simulink model "s_cd_hmc_v2"  (R2016b)
(part 2 of 43)

      mask prompts: io_dir "I/O direction"; io_delay "I/O delay"; sample_period "Sample period"; names "Bitfield names [msb...lsb]"; bitwidths "Bitfield widths"; bin_pts "Bitfield binary pts"; arith_types "Bitfield types, ufix=0, fix=1, bool=2"; sim_port "Provide sim input/output?"; show_format "Print format string?"
      mask help: A 32-bit software-accessible register. Can be divided into bitfields of varying widths and types using the fields in the block mask.
      mask init:
      | swreg_init(gcb)
      settings: AttributesFormatString=1input:uf32.0 = 32 bits
      mask TypeOptions io_dir: To Processor | From Processor
      mask Callback io_dir:
      | mask_enables = get_param(gcb, 'MaskEnables');
      | mask_names = get_param(gcb, 'MaskNames');
      | if strcmp(get_param(gcb, 'io_dir'), 'To Processor'),
      |     mask_enables{ismember(mask_names, 'sample_period')} = 'off';
      | else
      |     mask_enables{ismember(mask_names, 'sample_period')} = 'on';
      | end
      | set_param(gcb, 'MaskEnables', mask_enables);
  sync : Subsystem  Tag=xps:sw_reg  AncestorBlock=xps_library/software_register  mask(swreg){io_dir=To Processor, io_delay=0, sample_period=1, names=reg, bitwidths=1, bin_pts=0, arith_types=2, sim_port=on, show_format=on}
      mask prompts: io_dir "I/O direction"; io_delay "I/O delay"; sample_period "Sample period"; names "Bitfield names [msb...lsb]"; bitwidths "Bitfield widths"; bin_pts "Bitfield binary pts"; arith_types "Bitfield types, ufix=0, fix=1, bool=2"; sim_port "Provide sim input/output?"; show_format "Print format string?"
      mask help: A 32-bit software-accessible register. Can be divided into bitfields of varying widths and types using the fields in the block mask.
      mask init:
      | swreg_init(gcb)
      settings: AttributesFormatString=1output:b = 1 bits
      mask TypeOptions io_dir: To Processor | From Processor
      mask Callback io_dir:
      | mask_enables = get_param(gcb, 'MaskEnables');
      | mask_names = get_param(gcb, 'MaskNames');
      | if strcmp(get_param(gcb, 'io_dir'), 'To Processor'),
      |     mask_enables{ismember(mask_names, 'sample_period')} = 'off';
      | else
      |     mask_enables{ismember(mask_names, 'sample_period')} = 'on';
      | end
      | set_param(gcb, 'MaskEnables', mask_enables);
  sync_cnt : Subsystem  Tag=xps:sw_reg  AncestorBlock=xps_library/software_register  mask(swreg){io_dir=To Processor, io_delay=0, sample_period=1, names=reg, bitwidths=32, bin_pts=0, arith_types=0, sim_port=on, show_format=on}
      mask prompts: io_dir "I/O direction"; io_delay "I/O delay"; sample_period "Sample period"; names "Bitfield names [msb...lsb]"; bitwidths "Bitfield widths"; bin_pts "Bitfield binary pts"; arith_types "Bitfield types, ufix=0, fix=1, bool=2"; sim_port "Provide sim input/output?"; show_format "Print format string?"
      mask help: A 32-bit software-accessible register. Can be divided into bitfields of varying widths and types using the fields in the block mask.
      mask init:
      | swreg_init(gcb)
      settings: AttributesFormatString=1output:uf32.0 = 32 bits
      mask TypeOptions io_dir: To Processor | From Processor
      mask Callback io_dir:
      | mask_enables = get_param(gcb, 'MaskEnables');
      | mask_names = get_param(gcb, 'MaskNames');
      | if strcmp(get_param(gcb, 'io_dir'), 'To Processor'),
      |     mask_enables{ismember(mask_names, 'sample_period')} = 'off';
      | else
      |     mask_enables{ismember(mask_names, 'sample_period')} = 'on';
      | end
      | set_param(gcb, 'MaskEnables', mask_enables);
  sync_select : Subsystem  Tag=xps:sw_reg  AncestorBlock=xps_library/software register  mask(swreg){io_dir=From Processor, io_delay=0, sample_period=1, names=reg, bitwidths=2, bin_pts=0, arith_types=0, sim_port=on, show_format=on}
      mask prompts: io_dir "I/O direction"; io_delay "I/O delay"; sample_period "Sample period"; names "Bitfield names [msb...lsb]"; bitwidths "Bitfield widths"; bin_pts "Bitfield binary pts"; arith_types "Bitfield types, ufix=0, fix=1, bool=2"; sim_port "Provide sim input/output?"; show_format "Print format string?"
      mask help: A 32-bit software-accessible register. Can be divided into bitfields of varying widths and types using the fields in the block mask.
      mask init:
      | swreg_init(gcb)
      settings: AttributesFormatString=1input:uf2.0 = 2 bits
      mask TypeOptions io_dir: To Processor | From Processor
      mask Callback io_dir:
      | mask_enables = get_param(gcb, 'MaskEnables');
      | mask_names = get_param(gcb, 'MaskNames');
      | if strcmp(get_param(gcb, 'io_dir'), 'To Processor'),
      |     mask_enables{ismember(mask_names, 'sample_period')} = 'off';
      | else
      |     mask_enables{ismember(mask_names, 'sample_period')} = 'on';
      | end
      | set_param(gcb, 'MaskEnables', mask_enables);
  tl_cd0 : Subsystem  mask(timed_latch){n_bits_time=48-(fft_stages+8), n_bits_quantization=fft_stages+8, n_bits_counters=4}
      mask prompts: n_bits_time "Number bits in time to compare"; n_bits_quantization "Time offset from lsb"; n_bits_counters "Bits in status counters"
      mask help:
      | Latches load_value when armed and current_time matches requested time.
      | current_time should be in ADC samples.
      mask init:
      | set_param([gcb,'/status'], 'bitwidths', mat2str([1, repmat(n_bits_counters, 1, 2)]));
      mask Help:
      | When armed, will latch new value when current time matches the time
      | specified. The input time should be in samples and mask settings allow
      | a portion of this to be compared to cater for quantization. Arm and latch
      | counts allow the current state, pending and missed latch events to be
      | determined.
  tl_cd1 : Subsystem  mask(timed_latch){n_bits_time=48-(fft_stages+8), n_bits_quantization=fft_stages+8, n_bits_counters=4}
      mask prompts: n_bits_time "Number bits in time to compare"; n_bits_quantization "Time offset from lsb"; n_bits_counters "Bits in status counters"
      mask help:
      | Latches load_value when armed and current_time matches requested time.
      | current_time should be in ADC samples.
      mask init:
      | set_param([gcb,'/status'], 'bitwidths', mat2str([1, repmat(n_bits_counters, 1, 2)]));
      mask Help:
      | When armed, will latch new value when current time matches the time
      | specified. The input time should be in samples and mask settings allow
      | a portion of this to be compared to cater for quantization. Arm and latch
      | counts allow the current state, pending and missed latch events to be
      | determined.
  tx_metadata : Subsystem  Tag=xps:sw_reg  AncestorBlock=xps_library/software register  mask(swreg){io_dir=From Processor, io_delay=0, sample_period=1, names=[porttx board_id], bitwidths=16, bin_pts=0, arith_types=0, sim_port=on, show_format=on}
      mask prompts: io_dir "I/O direction"; io_delay "I/O delay"; sample_period "Sample period"; names "Bitfield names [msb...lsb]"; bitwidths "Bitfield widths"; bin_pts "Bitfield binary pts"; arith_types "Bitfield types, ufix=0, fix=1, bool=2"; sim_port "Provide sim input/output?"; show_format "Print format string?"
      mask help: A 32-bit software-accessible register. Can be divided into bitfields of varying widths and types using the fields in the block mask.
      mask init:
      | swreg_init(gcb)
      settings: AttributesFormatString=2 inputs:uf16.0,uf16.0 = 32 bits
      mask TypeOptions io_dir: To Processor | From Processor
      mask Callback io_dir:
      | mask_enables = get_param(gcb, 'MaskEnables');
      | mask_names = get_param(gcb, 'MaskNames');
      | if strcmp(get_param(gcb, 'io_dir'), 'To Processor'),
      |     mask_enables{ismember(mask_names, 'sample_period')} = 'off';
      | else
      |     mask_enables{ismember(mask_names, 'sample_period')} = 'on';
      | end
      | set_param(gcb, 'MaskEnables', mask_enables);
  valid80 : Subsystem  Tag=xps:sw_reg  AncestorBlock=xps_library/software_register  mask(swreg){io_dir=To Processor, io_delay=0, sample_period=1, names=reg, bitwidths=1, bin_pts=0, arith_types=2, sim_port=on, show_format=on}
      mask prompts: io_dir "I/O direction"; io_delay "I/O delay"; sample_period "Sample period"; names "Bitfield names [msb...lsb]"; bitwidths "Bitfield widths"; bin_pts "Bitfield binary pts"; arith_types "Bitfield types, ufix=0, fix=1, bool=2"; sim_port "Provide sim input/output?"; show_format "Print format string?"
      mask help: A 32-bit software-accessible register. Can be divided into bitfields of varying widths and types using the fields in the block mask.
      mask init:
      | swreg_init(gcb)
      settings: AttributesFormatString=1output:b = 1 bits
      mask TypeOptions io_dir: To Processor | From Processor
      mask Callback io_dir:
      | mask_enables = get_param(gcb, 'MaskEnables');
      | mask_names = get_param(gcb, 'MaskNames');
      | if strcmp(get_param(gcb, 'io_dir'), 'To Processor'),
      |     mask_enables{ismember(mask_names, 'sample_period')} = 'off';
      | else
      |     mask_enables{ismember(mask_names, 'sample_period')} = 'on';
      | end
      | set_param(gcb, 'MaskEnables', mask_enables);
  valid80_cnt : Subsystem  Tag=xps:sw_reg  AncestorBlock=xps_library/software_register  mask(swreg){io_dir=To Processor, io_delay=0, sample_period=1, names=reg, bitwidths=32, bin_pts=0, arith_types=0, sim_port=on, show_format=on}
      mask prompts: io_dir "I/O direction"; io_delay "I/O delay"; sample_period "Sample period"; names "Bitfield names [msb...lsb]"; bitwidths "Bitfield widths"; bin_pts "Bitfield binary pts"; arith_types "Bitfield types, ufix=0, fix=1, bool=2"; sim_port "Provide sim input/output?"; show_format "Print format string?"
      mask help: A 32-bit software-accessible register. Can be divided into bitfields of varying widths and types using the fields in the block mask.
      mask init:
      | swreg_init(gcb)
      settings: AttributesFormatString=1output:uf32.0 = 32 bits
      mask TypeOptions io_dir: To Processor | From Processor
      mask Callback io_dir:
      | mask_enables = get_param(gcb, 'MaskEnables');
      | mask_names = get_param(gcb, 'MaskNames');
      | if strcmp(get_param(gcb, 'io_dir'), 'To Processor'),
      |     mask_enables{ismember(mask_names, 'sample_period')} = 'off';
      | else
      |     mask_enables{ismember(mask_names, 'sample_period')} = 'on';
      | end
      | set_param(gcb, 'MaskEnables', mask_enables);
  tag scope: cnt_rst=global, dvalid=global, man_sys_rst=global, sync_select=global
  wires:
  Constant/1 -> port0/1(sim_1)
  port0/1(in_reg) -> Delay16/1
  Constant2/1 -> ip0/1(sim_1)
  ip0/1(in_reg) -> Delay15/1
  Constant3/1 -> forty_gbe/8(rx_overrun_ack)
  Constant4/1 -> forty_gbe/7(rx_ack)
  [gbe_rst] -> pipeline102/1(d)
  Delay15/1 -> forty_gbe/4(tx_dest_ip)
  Delay16/1 -> forty_gbe/5(tx_dest_port)
  Concat22/1 -> pipeline29/1(d)
  Concat3/1 -> pipeline27/1(d)
  phase0/1(in_initial) -> Reinterpret2/1
  delta_delay0/1(in_delta) -> Reinterpret1/1
  phase0/2(in_delta) -> Reinterpret3/1
  Reinterpret8/1 -> pipeline56/1(d)
  Reinterpret1/1 -> pipeline55/1(d)
  Reinterpret2/1 -> pipeline54/1(d)
  Reinterpret3/1 -> pipeline53/1(d)
  phase1/1(in_initial) -> Reinterpret5/1
  delta_delay1/1(in_delta) -> Reinterpret4/1
  phase1/2(in_delta) -> Reinterpret6/1
  Reinterpret4/1 -> pipeline51/1(d)
  Reinterpret5/1 -> pipeline50/1(d)
  Reinterpret6/1 -> pipeline49/1(d)
  Reinterpret7/1 -> pipeline52/1(d)
  delay0/1(in_initial) -> Reinterpret8/1
  delay1/1(in_initial) -> Reinterpret7/1
  Constant10/1 -> iptx_base/1(sim_1)
  Constant9/1 -> tx_metadata/1(sim_1)
  Constant13/1 -> tx_metadata/2(sim_2)
  iptx_base/1(in_reg) -> pipeline105/1(d)
  pipeline105/1(q) -> [tx_ip_base]
  tx_metadata/1(in_porttx) -> pipeline106/1(d)
  tx_metadata/2(in_board_id) -> pipeline107/1(d)
  pipeline106/1(q) -> [tx_port]
  pipeline107/1(q) -> [tx_board_id]
  edge_detect4/1(out) -> pipeline5/1(d)
  control1/6(in_cnt_rst) -> edge_detect1/1(in)
  edge_detect1/1(out) -> pipeline14/1(d)
  control1/3(in_gbe_rst) -> pipeline6/1(d)
  control1/1(in_sys_rst) -> pipeline3/1(d)
  pipeline3/1(q) -> [sys_rst]
  pipeline5/1(q) -> [clr_status]
  pipeline6/1(q) -> [gbe_rst]
  pipeline7/1(q) -> [gbe_txen]
  pipeline13/1(q) -> [tvg_adc_en]
  pipeline14/1(q) -> [cnt_rst]
  control1/5(in_tvg_adc) -> pipeline13/1(d)
  edge_detect2/1(out) -> pipeline38/1(d)
  pipeline38/1(q) -> [gbe_cnt_rst]
  control1/7(in_gbe_cnt_rst) -> edge_detect2/1(in)
  control1/4(in_gbe_txen) -> pipeline7/1(d)
  control1/2(in_status_clr) -> edge_detect4/1(in)
  pipeline43/1(q) -> [adc_snap_arm]
  control1/8(in_adc_snap_arm) -> pipeline43/1(d)
  control1/9(in_adc_snap_trig_select) -> pipeline39/1(d)
  pipeline39/1(q) -> [adc_snap_trig_source]
  [ld_val0] -> pipeline23/1(d)
  [clr_status] -> pipeline22/1(d)
  tl_cd0/6(time) -> Terminator16/1
  tl_cd0/3(sync_out) -> pipeline41/1(d)
  tl_cd0/4(dout) -> pipeline42/1(d)
  tl_cd0/5(dvalid) -> pipeline45/1(d)
  tl_cd0/1(value) -> pipeline46/1(d)
  tl_cd0/2(enable) -> pipeline48/1(d)
  cd_compensation0/5(parity_error) -> pipeline86/1(d)
  cd_compensation0/4(hmc_error) -> pipeline85/1(d)
  Constant6/1 -> Concat15/2
  Concat15/1 -> pipeline21/1(d)
  Counter2/1 -> pipeline31/1(d)
  Counter4/1 -> pipeline32/1(d)
  Counter9/1 -> pipeline33/1(d)
  Counter10/1 -> pipeline34/1(d)
  Counter11/1 -> pipeline35/1(d)
  Counter12/1 -> pipeline36/1(d)
  Counter14/1 -> pipeline40/1(d)
  Counter13/1 -> pipeline37/1(d)
  cd_compensation0/2(dout) -> pipeline83/1(d)
  cd_compensation0/1(sync_out) -> pipeline82/1(d)
  cd_compensation0/3(dvalid) -> pipeline84/1(d)
  hmc_error/1(sim_out) -> Terminator9/1
  [hmc_error] -> hmc_error/1(out_reg)
  hmc_parity/1(sim_out) -> Terminator11/1
  Logical3/1 -> hmc_parity/1(out_reg)
  Constant11/1 -> Delay10/1
  [valid80_local] -> Gateway Out19/1, pipeline58/1(d), pipeline61/1(d), pipeline62/1(d), pipeline63/1(d), pipeline64/1(d), pipeline65/1(d), pipeline66/1(d), pipeline60/1(d), pipeline59/1(d)
  [cd_in] -> pipeline25/1(d)
  bus_create1/1(bus_out) -> [cd_in]
  pipeline22/1(q) -> tl_cd0/1(rst)
  pipeline21/1(q) -> tl_cd0/2(current_time)
  pipeline23/1(q) -> tl_cd0/3(load_value)
  pipeline24/1(q) -> Gateway Out14/1, tl_cd0/4(sync_in)
  pipeline25/1(q) -> Gateway Out10/1, tl_cd0/5(din)
  pipeline26/1(q) -> Gateway Out11/1, tl_cd0/6(en)
  [sync80] -> Terminator7/1
  [valid80] -> Terminator10/1
  [valid80_cd] -> pipeline26/1(d)
  Gateway Out10/1 -> To Workspace6/1
  Gateway Out11/1 -> To Workspace7/1
  Gateway Out14/1 -> To Workspace8/1
  pipeline31/1(q) -> bus_create1/1(in1)
  pipeline32/1(q) -> bus_create1/2(in2)
  pipeline33/1(q) -> bus_create1/3(in3)
  pipeline34/1(q) -> bus_create1/4(in4)
  pipeline35/1(q) -> bus_create1/5(in5)
  pipeline36/1(q) -> bus_create1/6(in6)
  pipeline37/1(q) -> bus_create1/7(in7)
  pipeline40/1(q) -> bus_create1/8(in8)
  pipeline41/1(q) -> Gateway Out20/1, cd_compensation0/1(sync_in)
  pipeline42/1(q) -> cd_compensation0/2(din)
  pipeline45/1(q) -> Gateway Out21/1, cd_compensation0/3(en)
  pipeline48/1(q) -> cd_compensation0/5(load_val)
  pipeline46/1(q) -> cd_compensation0/4(delay_val)
  pipeline66/1(q) -> pipeline30/1(d)
  pipeline30/1(q) -> [valid80_cd]
  Constant24/1 -> forty_gbe/2(tx_data)
  Constant25/1 -> forty_gbe/3(tx_valid)
  Constant26/1 -> forty_gbe/6(tx_end_of_frame)
  pipeline27/1(q) -> [ld_val1]
  pipeline29/1(q) -> [ld_val0]
  pipeline49/1(q) -> Concat3/4
  pipeline50/1(q) -> Concat3/3
  pipeline51/1(q) -> Concat3/2
  pipeline52/1(q) -> Concat3/1
  pipeline53/1(q) -> Concat22/4
  pipeline54/1(q) -> Concat22/3
  pipeline55/1(q) -> Concat22/2
  pipeline56/1(q) -> Concat22/1
  bus_expand2/1(msb_out8) -> pipeline167/1(d)  "hmc_out9"
  bus_expand2/8(lsb_out1) -> pipeline73/1(d)  "hmc_out16"
  pipeline76/1(q) -> bus_expand2/1(bus_in)
  [cd_out_pol0] -> pipeline76/1(d)
  pipeline73/1(q) -> cd_out/8(in_d07)
  pipeline72/1(q) -> cd_out/7(in_d06)
  pipeline71/1(q) -> cd_out/6(in_d05)
  pipeline70/1(q) -> cd_out/5(in_d04)
  pipeline69/1(q) -> cd_out/4(in_d03)
  pipeline68/1(q) -> cd_out/3(in_d02)
  pipeline67/1(q) -> cd_out/2(in_d01)
  pipeline167/1(q) -> cd_out/1(in_d00)
  bus_expand2/7(out2) -> pipeline72/1(d)
  bus_expand2/5(out4) -> pipeline70/1(d)
  bus_expand2/4(out5) -> pipeline69/1(d)
  bus_expand2/6(out3) -> pipeline71/1(d)
  bus_expand2/3(out6) -> pipeline68/1(d)
  bus_expand2/2(out7) -> pipeline67/1(d)
  [cd_sync] -> pipeline79/1(d)
  pipeline75/1(q) -> cd_out/9(in_dvalid)
  pipeline74/1(q) -> cd_out/10(in_sync)
  pipeline82/1(q) -> Gateway Out13/1, [cd_sync]
  pipeline83/1(q) -> [cd_out_pol0], Gateway Out17/1
  pipeline84/1(q) -> Gateway Out16/1, [cd_dvalid]
  pipeline85/1(q) -> [hmc_error]
  pipeline86/1(q) -> [hmc_parity_pol0]
  [cd_dvalid] -> pipeline77/1(d)
  pipeline65/1(q) -> Counter14/2
  pipeline64/1(q) -> Counter13/2
  pipeline63/1(q) -> Counter12/2
  pipeline62/1(q) -> Counter11/2
  pipeline61/1(q) -> Counter10/2
  pipeline59/1(q) -> Counter4/2
  pipeline60/1(q) -> Counter9/2
  pipeline58/1(q) -> Counter2/2
  pipeline98/1(q) -> Counter2/1
  pipeline97/1(q) -> Counter4/1
  pipeline96/1(q) -> Counter9/1
  pipeline95/1(q) -> Counter10/1
  pipeline94/1(q) -> Counter11/1
  pipeline93/1(q) -> Counter12/1
  pipeline92/1(q) -> Counter13/1
  pipeline91/1(q) -> Counter14/1
  hmc_delay/1(sim_out) -> Terminator/1
  compute_delay/1(hmc_latency) -> pipeline99/1(d)
  pipeline99/1(q) -> hmc_delay/1(out_reg)
  [sync80_local] -> pipeline91/1(d), pipeline92/1(d), pipeline93/1(d), pipeline94/1(d), pipeline95/1(d), pipeline96/1(d), pipeline97/1(d), pipeline98/1(d)
  pipeline102/1(q) -> forty_gbe/1(rst)
  [cd_in] -> pipeline108/1(d)
  [cd_out_pol0] -> pipeline111/1(d)
  [cd_dvalid] -> pipeline110/1(d)
  [cd_sync] -> pipeline109/1(d)
  Constant1/1 -> pipeline112/1(d)
  [valid80_cd] -> pipeline104/1(d)
  [sync80_cd] -> pipeline103/1(d)
  pipeline103/1(q) -> compute_delay/1(cd_in_sync)
  pipeline104/1(q) -> compute_delay/2(cd_in_dvalid)
  pipeline108/1(q) -> compute_delay/3(cd_in)
  pipeline109/1(q) -> compute_delay/4(cd_out_sync)
  pipeline110/1(q) -> compute_delay/5(cd_out_dvalid)
  pipeline111/1(q) -> compute_delay/6(cd_out)
  pipeline112/1(q) -> compute_delay/7(trigger_threshold)
  cd_in_cnt_thresh/1(sim_out) -> Terminator2/1
  pipeline113/1(q) -> cd_in_cnt_thresh/1(out_reg)
  cd_out_cnt_thresh/1(sim_out) -> Terminator3/1
  pipeline114/1(q) -> cd_out_cnt_thresh/1(out_reg)
  compute_delay/3(cd_out_count_sync_threshold) -> pipeline114/1(d)
  compute_delay/2(cd_in_count_sync_threshold) -> pipeline113/1(d)
  Constant5/1 -> sync_select/1(sim_1)
  [time80] -> Terminator4/1
  Constant27/1 -> Concat15/1
  pipeline2/1(q) -> bus_expand3/1(bus_in)
  [cd_in] -> pipeline2/1(d)
  Gateway Out45/1 -> To Workspace2/1
  Gateway Out46/1 -> To Workspace3/1
  Gateway Out47/1 -> To Workspace5/1
  Gateway Out48/1 -> To Workspace11/1
  Gateway Out49/1 -> To Workspace12/1
  Gateway Out50/1 -> To Workspace13/1
  Gateway Out51/1 -> To Workspace14/1
  bus_expand3/1(msb_out8) -> Gateway Out43/1
  bus_expand3/2(out7) -> Gateway Out45/1
  bus_expand3/3(out6) -> Gateway Out46/1
  bus_expand3/4(out5) -> Gateway Out47/1
  bus_expand3/5(out4) -> Gateway Out48/1
  bus_expand3/6(out3) -> Gateway Out49/1
  bus_expand3/7(out2) -> Gateway Out50/1
  bus_expand3/8(lsb_out1) -> Gateway Out51/1
  Gateway Out43/1 -> To Workspace4/1
  [cd_out_pol0] -> bus_expand4/1(bus_in)
  Gateway Out3/1 -> To Workspace16/1
  Gateway Out5/1 -> To Workspace17/1
  Gateway Out6/1 -> To Workspace18/1
  Gateway Out7/1 -> To Workspace19/1
  bus_expand4/1(msb_out8) -> Gateway Out2/1
  bus_expand4/2(out7) -> Gateway Out3/1
  bus_expand4/3(out6) -> Gateway Out5/1
  bus_expand4/4(out5) -> Gateway Out6/1
  bus_expand4/5(out4) -> Gateway Out7/1
  bus_expand4/6(out3) -> Gateway Out8/1
  bus_expand4/7(out2) -> Gateway Out9/1
  bus_expand4/8(lsb_out1) -> Gateway Out12/1
  Gateway Out2/1 -> To Workspace21/1
  Gateway Out12/1 -> To Workspace23/1
  Gateway Out9/1 -> To Workspace22/1
  Gateway Out8/1 -> To Workspace20/1
  [sync80_local] -> Gateway Out18/1, pipeline8/1(d)
  pipeline8/1(q) -> pipeline9/1(d)
  pipeline9/1(q) -> [sync80_cd]
  [sync80_cd] -> pipeline24/1(d)
  Gateway Out13/1 -> To Workspace15/1
  Gateway Out16/1 -> To Workspace24/1
  Gateway Out17/1 -> To Workspace25/1
  Gateway Out18/1 -> To Workspace26/1
  Gateway Out19/1 -> To Workspace27/1
  Constant7/1 -> To Workspace28/1, delay0/1(sim_1)
  Gateway Out20/1 -> To Workspace29/1
  Gateway Out21/1 -> To Workspace30/1
  sync_select/1(in_reg) -> pipeline4/1(d)
  pipeline4/1(q) -> [sync_select]
  dvalid/1(in_reg) -> pipeline16/1(d)
  pipeline16/1(q) -> [dvalid]
  man_sync/1(in_reg) -> pipeline17/1(d)
  Constant17/1 -> Delay/1
  sync/1(sim_out) -> To Workspace102/1
  pipeline115/1(q) -> Register1/3, Register1/1
  pipeline20/1(q) -> Register1/2
  sync_cnt/1(sim_out) -> To Workspace104/1
  Counter1/1 -> pipeline129/1(d)
  pipeline129/1(q) -> sync_cnt/1(out_reg)
  pipeline131/1(q) -> sync/1(out_reg)
  Register1/1 -> pipeline131/1(d)
  pipeline116/1(q) -> Counter1/1
  pipeline101/1(q) -> Counter1/2
  [man_sys_rst] -> edge_detect11/1
  [sync80_local] -> edge_detect9/1
  valid80/1(sim_out) -> To Workspace38/1
  pipeline90/1(q) -> Register2/3, Register2/1
  pipeline47/1(q) -> Register2/2
  valid80_cnt/1(sim_out) -> To Workspace39/1
  Counter3/1 -> pipeline28/1(d)
  pipeline28/1(q) -> valid80_cnt/1(out_reg)
  pipeline44/1(q) -> valid80/1(out_reg)
  Register2/1 -> pipeline44/1(d)
  pipeline100/1(q) -> Counter3/1
  pipeline80/1(q) -> Counter3/2
  [man_sys_rst] -> edge_detect6/1
  [valid80_local] -> edge_detect5/1
  edge_detect5/1 -> pipeline90/1(d), pipeline80/1(d)
  edge_detect6/1 -> pipeline100/1(d), pipeline47/1(d)
  edge_detect9/1 -> pipeline101/1(d), pipeline115/1(d)
  edge_detect11/1 -> pipeline20/1(d), pipeline116/1(d)
  pipeline17/1(q) -> [man_sync]
  pipeline117/1(q) -> [man_sys_rst]
  Constant18/1 -> man_sys_rst/1(sim_1)
  man_sys_rst/1(in_reg) -> pipeline117/1(d)
  Delay/1 -> man_sync/1(sim_1)
  Delay10/1 -> dvalid/1(sim_1)
  bus_expand1/8(lsb_out1) -> pipeline176/1(d)  "hmc_out16"
  pipeline222/1(q) -> bus_expand1/1(bus_in)
  [cd_in] -> pipeline222/1(d)
  pipeline176/1(q) -> cd_in/8(in_d07)
  pipeline175/1(q) -> cd_in/7(in_d06)
  pipeline172/1(q) -> cd_in/6(in_d05)
  pipeline171/1(q) -> cd_in/5(in_d04)
  pipeline170/1(q) -> cd_in/4(in_d03)
  pipeline169/1(q) -> cd_in/3(in_d02)
  pipeline168/1(q) -> cd_in/2(in_d01)
  bus_expand1/7(out2) -> pipeline175/1(d)
  bus_expand1/5(out4) -> pipeline171/1(d)
  bus_expand1/4(out5) -> pipeline170/1(d)
  bus_expand1/6(out3) -> pipeline172/1(d)
  bus_expand1/3(out6) -> pipeline169/1(d)
  bus_expand1/2(out7) -> pipeline168/1(d)
  pipeline19/1(q) -> pipeline178/1(d), Logical/1
  pipeline178/1(q) -> cd_in/9(in_dvalid)
  pipeline177/1(q) -> cd_in/10(in_sync)
  bus_expand1/1(msb_out8) -> pipeline87/1(d)
  pipeline87/1(q) -> cd_in/1(in_d00)
  [valid80_cd] -> pipeline19/1(d)
  [sync80_cd] -> pipeline15/1(d)
  pipeline15/1(q) -> pipeline177/1(d), pipeline57/1(d), Logical/2
  pipeline57/1(q) -> cd_in/12(trig)
  pipeline18/1(q) -> cd_in/11(we)
  Logical/1 -> pipeline18/1(d)
  pipeline81/1(q) -> cd_out/12(trig)
  pipeline78/1(q) -> cd_out/11(we)
  Logical1/1 -> pipeline78/1(d)
  pipeline79/1(q) -> pipeline81/1(d), Logical1/2, pipeline74/1(d)
  pipeline77/1(q) -> pipeline75/1(d), Logical1/1
  Counter5/1 -> Gateway Out27/1, Relational1/1
  Constant32/1 -> Relational1/2
  Gateway Out15/1 -> To Workspace42/1
  Gateway Out1/1 -> To Workspace1/1
  Delay1/1 -> Delay3/1
  Delay7/1 -> Delay12/1
  Gateway Out4/1 -> To Workspace10/1
  Delay9/1 -> Delay13/1
  [valid80] -> Terminator1/1
  Mux1/1 -> edge_detect12/1
  Delay3/1 -> Gateway Out28/1, Mux2/2
  [sync_select] -> Mux2/1, Gateway Out25/1, Mux1/1
  [dvalid] -> edge_detect13/1, Logical16/3
  Register3/1 -> Delay8/1, Gateway Out29/1, Inverter3/1
  Delay6/1 -> Delay17/1
  Delay8/1 -> Delay1/1
  Gateway Out24/1 -> To Workspace35/1
  Gateway Out25/1 -> To Workspace36/1
  Gateway Out26/1 -> To Workspace37/1
  Gateway Out27/1 -> To Workspace40/1
  edge_detect3/1 -> Counter5/1
  Mux2/1 -> [valid80_local], Gateway Out15/1
  Gateway Out28/1 -> To Workspace41/1
  Delay4/1 -> Mux2/3
  Relational1/1 -> Mux1/3, Gateway Out24/1
  Delay17/1 -> Gateway Out26/1, Mux1/2
  edge_detect/1 -> Delay9/1
  Counter6/1 -> Slice1/1, Gateway Out31/1
  Slice1/1 -> Register3/3, Register3/1, Gateway Out30/1, edge_detect/1
  Gateway Out29/1 -> To Workspace9/1
  Gateway Out30/1 -> To Workspace33/1
  Gateway Out31/1 -> To Workspace34/1
  edge_detect8/1 -> Counter6/1
  Inverter3/1 -> Logical2/2
  edge_detect10/1 -> Register3/2
  Logical16/1 -> Register4/3, Delay11/1, Gateway Out32/1, Register4/1
  edge_detect13/1 -> Gateway Out33/1, Register4/2
  Gateway Out32/1 -> To Workspace43/1
  Gateway Out33/1 -> To Workspace44/1
  Gateway Out34/1 -> To Workspace45/1
  Logical2/1 -> Counter6/2
  Delay2/1 -> Counter5/2
  Delay5/1 -> Relational1/3
  Register4/1 -> edge_detect10/1, Delay7/1, Delay5/1, Delay2/1, Logical2/1, edge_detect3/1, Gateway Out34/1, edge_detect8/1
  edge_detect12/1 -> [sync80_local], Gateway Out1/1
  [man_sync] -> Mux1/4
  Delay11/1 -> Mux2/4
  [hmc_post] -> Logical16/1
  [hmc_init] -> Logical16/2
  Delay12/1 -> Gateway Out4/1, Delay4/1
  [ld_val0] -> pipeline89/1(d)
  [clr_status] -> pipeline88/1(d)
  tl_cd1/6(time) -> Terminator5/1
  tl_cd1/3(sync_out) -> pipeline121/1(d)
  tl_cd1/4(dout) -> pipeline122/1(d)
  tl_cd1/5(dvalid) -> pipeline123/1(d)
  tl_cd1/1(value) -> pipeline124/1(d)
  tl_cd1/2(enable) -> pipeline125/1(d)
  cd_compensation1/5(parity_error) -> pipeline132/1(d)
  cd_compensation1/4(hmc_error) -> pipeline130/1(d)
  Constant19/1 -> Concat1/2
  Concat1/1 -> pipeline11/1(d)
  cd_compensation1/2(dout) -> pipeline127/1(d)
  cd_compensation1/1(sync_out) -> pipeline126/1(d)
  cd_compensation1/3(dvalid) -> pipeline128/1(d)
  [cd_in] -> pipeline119/1(d)
  pipeline88/1(q) -> tl_cd1/1(rst)
  pipeline11/1(q) -> tl_cd1/2(current_time)
  pipeline89/1(q) -> tl_cd1/3(load_value)
  pipeline118/1(q) -> tl_cd1/4(sync_in)
  pipeline119/1(q) -> tl_cd1/5(din)
  pipeline120/1(q) -> tl_cd1/6(en)
  [valid80_cd] -> pipeline120/1(d)
  pipeline121/1(q) -> cd_compensation1/1(sync_in)
  pipeline122/1(q) -> cd_compensation1/2(din)
  pipeline123/1(q) -> cd_compensation1/3(en)
  pipeline125/1(q) -> cd_compensation1/5(load_val)
  pipeline124/1(q) -> cd_compensation1/4(delay_val)
  pipeline126/1(q) -> Gateway Out22/1, Terminator8/1
  pipeline127/1(q) -> Gateway Out35/1, [cd_out_pol1]
  pipeline128/1(q) -> Gateway Out23/1, Terminator12/1
  pipeline132/1(q) -> [hmc_parity_pol1]
  Constant16/1 -> Concat1/1
  [sync80_cd] -> pipeline118/1(d)
  pipeline130/1(q) -> Terminator6/1
  [hmc_parity_pol0] -> Logical3/1
  [hmc_parity_pol1] -> Logical3/2
  Gateway Out22/1 -> To Workspace31/1
  Gateway Out23/1 -> To Workspace32/1
  Gateway Out35/1 -> To Workspace46/1
  bus_expand5/1(msb_out8) -> pipeline133/1(d)  "hmc_out9"
  bus_expand5/8(lsb_out1) -> pipeline140/1(d)  "hmc_out16"
  pipeline143/1(q) -> bus_expand5/1(bus_in)
  [cd_out_pol1] -> pipeline143/1(d)
  pipeline140/1(q) -> cd_out1/8(in_d07)
  pipeline139/1(q) -> cd_out1/7(in_d06)
  pipeline138/1(q) -> cd_out1/6(in_d05)
  pipeline137/1(q) -> cd_out1/5(in_d04)
  pipeline136/1(q) -> cd_out1/4(in_d03)
  pipeline135/1(q) -> cd_out1/3(in_d02)
  pipeline134/1(q) -> cd_out1/2(in_d01)
  pipeline133/1(q) -> cd_out1/1(in_d00)
  bus_expand5/7(out2) -> pipeline139/1(d)
  bus_expand5/5(out4) -> pipeline137/1(d)
  bus_expand5/4(out5) -> pipeline136/1(d)
  bus_expand5/6(out3) -> pipeline138/1(d)
  bus_expand5/3(out6) -> pipeline135/1(d)
  bus_expand5/2(out7) -> pipeline134/1(d)
  [cd_sync] -> pipeline146/1(d)
  pipeline142/1(q) -> cd_out1/9(in_dvalid)
  pipeline141/1(q) -> cd_out1/10(in_sync)
  [cd_dvalid] -> pipeline144/1(d)
  [cd_out_pol1] -> bus_expand6/1(bus_in)
  Gateway Out38/1 -> To Workspace47/1
  Gateway Out40/1 -> To Workspace49/1
  bus_expand6/1(msb_out8) -> Gateway Out37/1
  bus_expand6/2(out7) -> Gateway Out38/1
  bus_expand6/3(out6) -> Gateway Out39/1
  bus_expand6/4(out5) -> Gateway Out40/1
  bus_expand6/5(out4) -> Gateway Out41/1
  bus_expand6/6(out3) -> Gateway Out42/1
  bus_expand6/7(out2) -> Gateway Out44/1
  bus_expand6/8(lsb_out1) -> Gateway Out36/1
  Gateway Out37/1 -> To Workspace52/1
  Gateway Out44/1 -> To Workspace53/1
  Gateway Out42/1 -> To Workspace51/1
  pipeline147/1(q) -> cd_out1/12(trig)
  pipeline145/1(q) -> cd_out1/11(we)
  Logical4/1 -> pipeline145/1(d)
  pipeline146/1(q) -> pipeline141/1(d), Logical4/2, pipeline147/1(d)
  pipeline144/1(q) -> Logical4/1, pipeline142/1(d)
  Gateway Out39/1 -> To Workspace48/1
  Gateway Out41/1 -> To Workspace50/1
  Gateway Out36/1 -> To Workspace54/1
  Delay13/1 -> Delay6/1
